simulink model "reference_2024"  (R2021a)
settings: Solver=ode23tb  StartTime=0.0  StopTime=20  RelTol=1e-4
libraries: spsSampleandHoldLib x2, spsExcitationSystemLib x1, spsHydraulicTurbineandGovernorLib x1, spsSynchronousMachinepuStandardLib x1, spspowerguiLib x1
settings Model: ExtModeTrigMode=oneshot  ExtModeArmWhenConnect=off  ExtModeAutoUpdateStatusClock=off  Creator=The MathWorks, Inc.  LastModifiedBy=Chen
settings SolverCC: AlgebraicLoopSolver=TrustRegion
settings DataIOCC: SaveFormat=Array  ReturnWorkspaceOutputs=off  SignalLoggingName=sigsOut
settings OptimizationCC: BlockReduction=off  BooleanDataType=off  ExpressionDepthLimit=2147483647  InitFltsAndDblsToZero=on  EfficientMapNaN2IntZero=off  LifeSpan=inf
settings DebuggingCC: UnderspecifiedInitializationDetection=Classic  MergeDetectMultiDrivingBlocksExec=none  CheckExecutionContextPreStartOutputMsg=on  SignalResolutionControl=TryResolveAllWithWarning  MultiTaskDSMMsg=warning  MultiTaskCondExecSysMsg=none  SigSpecEnsureSampleTimeMsg=none  FcnCallInpInsideContextMsg=warning  StateNameClashWarn=warning  SFUnexpectedBacktrackingDiag=warning  SFNoUnconditionalDefaultTransitionDiag=warning  SFExecutionAtInitializationDiag=none  ArithmeticOperatorsInVariantConditions=warning
settings HardwareCC: ProdBitPerPointer=32  ProdBitPerSizeT=32  ProdBitPerPtrDiffT=32  ProdLargestAtomicFloat=None  ProdIntDivRoundTo=Undefined  ProdEndianess=Unspecified  ProdWordSize=32  ProdHWDeviceType=32-bit Generic  TargetUnknown=on
settings ModelReferenceCC: PropagateSignalLabelsOutOfModel=off
settings SFSimCC: SimUseLocalCustomCode=off  CustomCodeUndefinedFunction=UseInterfaceOnly
settings RTWCC: RTWUseLocalCustomCode=off
settings CodeAppCC: StateflowObjectComments=on
settings GRTTargetCC: TargetLangStandard=C89/C90 (ANSI)  CombineOutputUpdateFcns=off  GRTInterface=on
settings ConfigComp: CovMetricSettings=dw  CovSaveCumulativeToWorkspaceVar=on  CovSaveSingleToWorkspaceVar=on  CovExternalEMLEnable=off  CovSFcnEnable=off
settings SimscapeCC: SimscapeNormalizeSystem=off

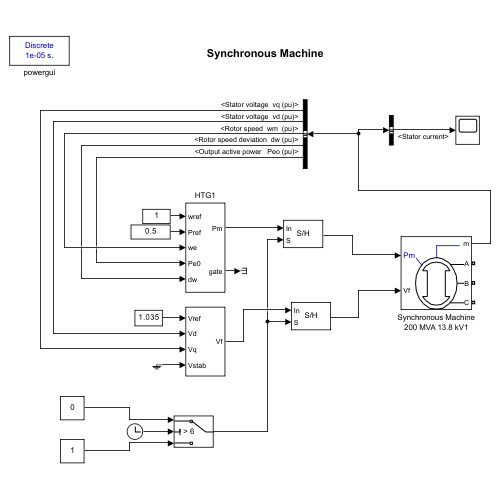
[thumbnail: Simulink's stored preview of the top-level diagram]
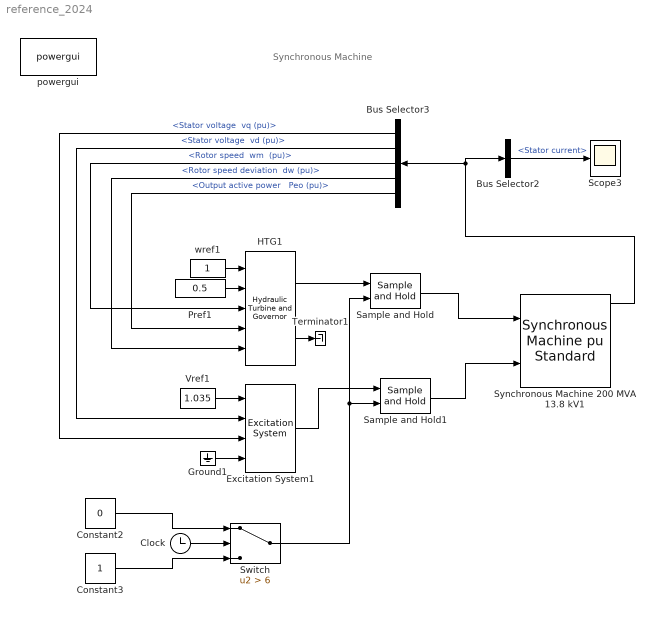
== system reference_2024 ==
  note: Synchronous Machine
  Bus Selector2 : BusSelector  OutputSignals=Stator current
  Bus Selector3 : BusSelector  OutputSignals="dq0 components.Stator voltage  vq (pu),dq0 components.Stator voltage  vd (pu),Mechanical.Rotor speed  wm  (pu),Mechanical.Rotor speed deviation  dw (pu),Output active power   Peo (pu)"
  Clock : Clock
  Constant2 : Constant  Value=0
  Constant3 : Constant
  Excitation System1 : spsExcitationSystemLib/Excitation System  tr=20e-3  reg=[ 300, 0.001 ]  exc=[ 1, 0 ]  tgr=[ 0, 0 ]  damp=[ 0.001, 0.1 ]  sat=[ 0, 0 ]  lim=[ -11.5, 11.5, 0 ]  v0=[1,1.29071]
  Ground1 : Ground
  HTG1 : spsHydraulicTurbineandGovernorLib/Hydraulic Turbine and Governor  sm="[ 10/3  0.07 ]"  gate="[  0.01  0.97518  -0.1  0.1 ]"  reg="[  0.05  1.163  0.105  0  0.01  ]"  hyd="[  0  2.67  ]"  dref=0  po=0.5
  Pref1 : Constant  Value=0.5
  Sample and Hold : spsSampleandHoldLib/Sample and Hold  ic=0  Ts=0
  Sample and Hold1 : spsSampleandHoldLib/Sample and Hold  ic=0  Ts=0
  Scope3 : Scope
  Switch : Switch  Criteria=u2 > Threshold  Threshold=6
  Synchronous Machine 200 MVA 13.8 kV1 : spsSynchronousMachinepuStandardLib/Synchronous Machine pu Standard  PresetModel=No  MechanicalLoad=Mechanical power Pm  ShowDetailedParameters=on  RotorType=Round  Units=per unit standard parameters  MeasurementBus=off  NominalParameters="[ 200E6  13800   50 ]"  Reactances1=[ 2.08, 0.296, 0.20, 1.62,0.474, 0.20, 0.15 ]  Reactances2=[ 1.305, 0.296, 0.252, 0.474, 0.243, 0.18 ]  dAxisTimeConstants=Open-circuit  qAxisTimeConstants=Open-circuit  TimeConstants1=[]  TimeConstants2=[ 9.3, 0.05, 0.8,0.07 ]  TimeConstants3=[]  TimeConstants4=[]  TimeConstants5=[ 1.01, 0.053, 0.1 ]  TimeConstants6=[ 9.3, 0.05, 0.8,0.07 ]  TimeConstants7=[]  TimeConstants8=[]  StatorResistance=2.05e-3  Mechanical=[ 3.3 0 2]  PolePairs=2  InitialConditions=[0 -94.2826 0.750185 0.750185 0.750185 -24.943 -144.943 95.057 1.29071]  SetSaturation=off  Saturation=[0.6404,0.7127,0.8441,0.9214,0.9956,1.082,1.19,1.316,1.457;0.7,0.7698,0.8872,0.9466,0.9969,1.046,1.1,1.151,1.201]  LoadFlowParameters=[1 150000000 0 0]  TsPowergui=0  TsBlock=-1  IterativeModel=Trapezoidal non iterative  IterativeDiscreteModel=Trapezoidal non iterative  BusType=PQ  Pref=100000000  Qref=20000000  Qmin=-Inf  Qmax=Inf  PLF=0  QLF=0
  Terminator1 : Terminator
  Vref1 : Constant  Value=1.035
  powergui : spspowerguiLib/powergui  Priority=2  SimulationMode=Discrete  SampleTime=10e-6  frequency=60  Iterations=50  frequencyindice=50  Pbase=100e6  ErrMax=0.0001  UnitsV=kV  UnitsW=MW  buscounter=0  FunctionMessages=off  echomessages=off  EnableUseOfTLC=off  CurrentSourceSwitches=off  DisableSnubberDevices=off  DisableRonSwitches=off  DisableVfSwitches=off  DisplayEquations=off  AutomaticDiscreteSolvers=off  SolverType=Tustin  Interpol=off  ExternalGateDelay=off  methode=off  Ts=0  x0status=blocks  SPID=on  SwTol=0  HookPort=off  NonlinearTolerance=1e-4  nMaxIteration=100  ContinueOnMaxIteration=off  RestoreLinks=warning  ResistiveCurrentMeasurement=off  Frange=logspace(0,3,50)  Ylog=off  Xlog=off  ShowGrid=off  save=off  variable=ZData  structure=0  ZoomFFT=on  StartTime=0.0  cycles=2  DisplayStyle=off  fundamental=60  FreqAxis=off  MaxFrequency=1000  frequencyindicesteady=1  RmsSteady=1  display=off
  wref1 : Constant
  wires:
  Bus Selector3/3 -> HTG1/3  "<Rotor speed  wm  (pu)>"
  Bus Selector3/5 -> HTG1/4  "<Output active power   Peo (pu)>"
  Bus Selector3/2 -> Excitation System1/2  "<Stator voltage  vd (pu)>"
  Bus Selector2/1 -> Scope3/1  "<Stator current>"
  HTG1/2 -> Terminator1/1
  Bus Selector3/1 -> Excitation System1/3  "<Stator voltage  vq (pu)>"
  Pref1/1 -> HTG1/2
  HTG1/1 -> Sample and Hold/1
  Ground1/1 -> Excitation System1/4
  Bus Selector3/4 -> HTG1/5  "<Rotor speed deviation  dw (pu)>"
  Vref1/1 -> Excitation System1/1
  Synchronous Machine 200 MVA 13.8 kV1/1 -> Bus Selector2/1, Bus Selector3/1
  wref1/1 -> HTG1/1
  Excitation System1/1 -> Sample and Hold1/1
  Sample and Hold/1 -> Synchronous Machine 200 MVA 13.8 kV1/1
  Sample and Hold1/1 -> Synchronous Machine 200 MVA 13.8 kV1/2
  Switch/1 -> Sample and Hold/2, Sample and Hold1/2
  Clock/1 -> Switch/2
  Constant2/1 -> Switch/1
  Constant3/1 -> Switch/3
